simulink model "Three_ph_T_DDparam1"  (R2024b)
settings: Solver=VariableStepAuto  StartTime=0.0  StopTime=10  RelTol=1e-3
values from neighbouring files (symbols this model uses):
  Lp = 0    [Three_ph_TFimptest_DD.m]
  Ls = 0.084225    [Three_ph_TFimptest_DD.m]
  P = 200e6    (= 200000000)    [Three_ph_TFimptest_DD.m]
  Rp = 4.3218    [Three_ph_TFimptest_DD.m]
  Rs = 0.7938    [Three_ph_TFimptest_DD.m]
  V = 20e3    (= 20000)    [Three_ph_TFimptest_DD.m]
  V1 = 2 * V2    (= 20000)    [Three_ph_TFimptest_DD.m]
  V2 = 1e4    (= 10000)    [Three_ph_TFimptest_DD.m]
undefined symbols (not defined in the file or in its folder): D1, Delta
libraries: spsGroundLib x7, spsCurrentMeasurementLib x6, spsACVoltageSourceLib x3, spsLinearTransformerLib x3, spsVoltageMeasurementLib x3, spsThreePhaseVIMeasurementLib x2, spsThreePhaseTransformerTwoWindingsLib x1, spsThreePhaseProgrammableVoltageSourceLib x1, spspowerguiLib x1
settings Model: PacingRate=0.100000  Creator=salsarayreh  LastModifiedBy=PC1

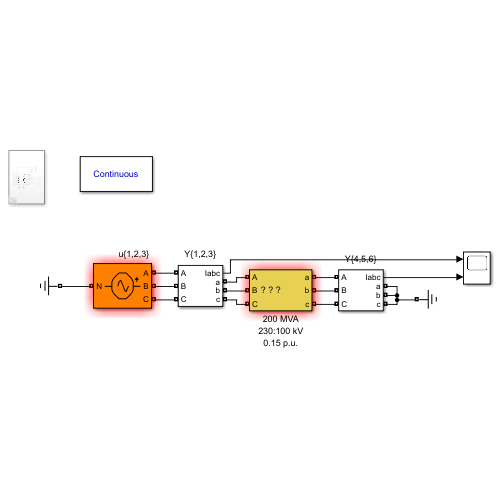
[thumbnail: Simulink's stored preview of the top-level diagram]
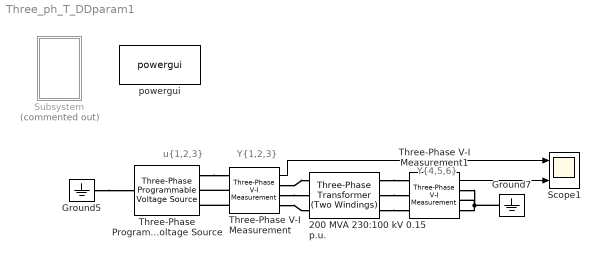
== system Three_ph_T_DDparam1 ==
  note: Y{4,5,6}
  note: Y{1,2,3}
  note: u{1,2,3}
  200 MVA 230:100 kV 0.15 p.u. : spsThreePhaseTransformerTwoWindingsLib/Three-Phase Transformer (Two Windings)  Winding1Connection=Delta (D1)  Winding2Connection=Delta (D1)  CoreType=Three single-phase transformers  SetSaturation=off  Hysteresis=off  DataFile='hysteresis'  SetInitialFlux=off  Measurements=All measurements (V I Fluxes)  UNITS=SI  NominalPower=[P , 50]  Winding1=[V1 Rp Lp ]  Winding2=[V2 Rs Ls]  Rm=Rm  Lm=Lm  L0=0.5  Saturation=[0 0;9.3114 683.7;785.26 875.13]  InitialFluxes=[-1.03850588171453 0.527233233676132 0.511272648041703]  BreakLoop=off  DiscreteSolver=Trapezoidal iterative  DataType=on  TransfoNumber=0
  Ground5 : spsGroundLib/Ground  LConnTagsString=a
  Ground7 : spsGroundLib/Ground  LConnTagsString=a
  Scope1 : Scope  NumInputPorts=2
  Subsystem : Subsystem  Commented=on
  Three-Phase Programmable Voltage Source : spsThreePhaseProgrammableVoltageSourceLib/Three-Phase Programmable Voltage Source  PositiveSequence="[V  0  50]"  VariationEntity=Amplitude  VariationType=Step  VariationTypeAlt=Step  VariationStep=-0.1  VariationRate=10  VariationMagnitude=0.3  VariationFrequency=2  VariationTiming="[0  0.14] + 1.5"  VariationPhaseA=off  Amplitudes=[1 0.8 1.2 1.0]  TimeValues=[0 0.1 0.15 0.2]  HarmonicGeneration=off  HarmonicA="[2 0.10  0  2]"  HarmonicB="[2  0  35 2]"  Timing="[1.2  99]"  BusType=swing  Pref=0  Qref=0  Qmin=-inf  Qmax=inf
  Three-Phase V-I Measurement : spsThreePhaseVIMeasurementLib/Three-Phase V-I Measurement  VoltageMeasurement=no  SetLabelV=off  LabelV=Vabc  Vpu=off  VpuLL=off  CurrentMeasurement=yes  SetLabelI=off  LabelI=Iabc  Ipu=off  Pbase=100e6  Vbase=500e3  OutputType=Complex  PhasorSimulation=off  PSBequivalent=0
  Three-Phase V-I Measurement1 : spsThreePhaseVIMeasurementLib/Three-Phase V-I Measurement  VoltageMeasurement=no  SetLabelV=off  LabelV=Vabc  Vpu=off  VpuLL=off  CurrentMeasurement=yes  SetLabelI=off  LabelI=Iabc  Ipu=off  Pbase=100e6  Vbase=500e3  OutputType=Complex  PhasorSimulation=off  PSBequivalent=0
  powergui : spspowerguiLib/powergui  Priority=1  SimulationMode=Continuous  SampleTime=50e-6  frequency=60  Iterations=50  frequencyindice=50  Pbase=100e6  ErrMax=1e-4  UnitsV=kV  UnitsW=MW  buscounter=0  FunctionMessages=off  echomessages=off  EnableUseOfTLC=off  CurrentSourceSwitches=off  DisableSnubberDevices=off  DisableRonSwitches=off  DisableVfSwitches=off  DisplayEquations=off  AutomaticDiscreteSolvers=off  SolverType=Tustin/Backward Euler (TBE)  Interpol=off  ExternalGateDelay=off  methode=off  Ts=100  x0status=blocks  SPID=on  SwTol=0  HookPort=off  NonlinearTolerance=1e-4  nMaxIteration=100  ContinueOnMaxIteration=off  RestoreLinks=warning  ResistiveCurrentMeasurement=off  Frange=[0:2:500]  Ylog=off  Xlog=on  ShowGrid=off  save=off  variable=ZData  structure=0  ZoomFFT=off  StartTime=0.0  cycles=1  DisplayStyle=1  fundamental=60  FreqAxis=off  MaxFrequency=1000  frequencyindicesteady=1  RmsSteady=1  display=off
  wires:
  Three-Phase V-I Measurement1/1 -> Scope1/2
  Three-Phase V-I Measurement/1 -> Scope1/1
  connections:
  Ground5/LConn1 -- Three-Phase Programmable Voltage Source/LConn1
  200 MVA 230:100 kV 0.15 p.u./RConn1 -- Three-Phase V-I Measurement1/LConn1
  200 MVA 230:100 kV 0.15 p.u./RConn2 -- Three-Phase V-I Measurement1/LConn2
  200 MVA 230:100 kV 0.15 p.u./RConn3 -- Three-Phase V-I Measurement1/LConn3
  Ground7/LConn1 -- Three-Phase V-I Measurement1/RConn1 -- Three-Phase V-I Measurement1/RConn2 -- Three-Phase V-I Measurement1/RConn3
  Three-Phase V-I Measurement/RConn2 -- 200 MVA 230:100 kV 0.15 p.u./LConn2
  Three-Phase V-I Measurement/RConn3 -- 200 MVA 230:100 kV 0.15 p.u./LConn3
  Three-Phase V-I Measurement/RConn1 -- 200 MVA 230:100 kV 0.15 p.u./LConn1
  Three-Phase V-I Measurement/LConn3 -- Three-Phase Programmable Voltage Source/RConn3
  Three-Phase V-I Measurement/LConn2 -- Three-Phase Programmable Voltage Source/RConn2
  Three-Phase Programmable Voltage Source/RConn1 -- Three-Phase V-I Measurement/LConn1

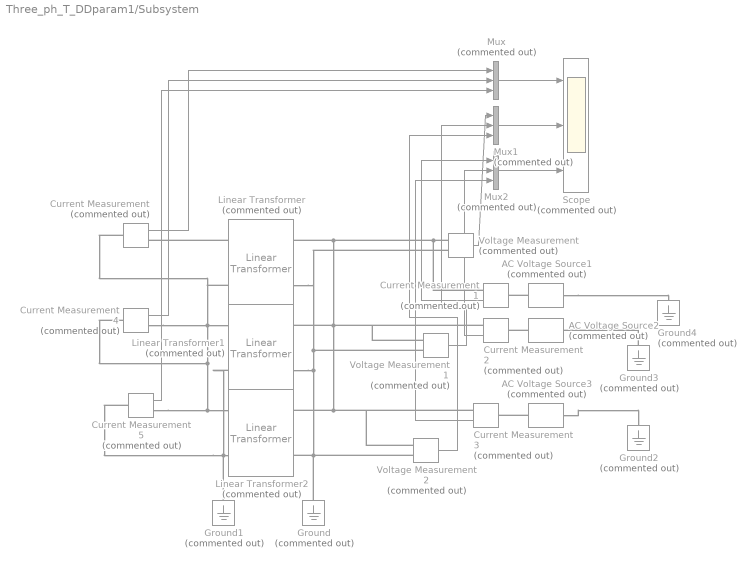
== system Three_ph_T_DDparam1/Subsystem ==
  AC Voltage Source1 : spsACVoltageSourceLib/AC Voltage Source  Commented=on  Amplitude=1  Phase=0  Frequency=50  SampleTime=0  Measurements=None  BusType=swing  Pref=10e3  Qref=0  Qmin=-inf  Qmax=+inf
  AC Voltage Source2 : spsACVoltageSourceLib/AC Voltage Source  Commented=on  Amplitude=1  Phase=-120  Frequency=50  SampleTime=0  Measurements=None  BusType=swing  Pref=10e3  Qref=0  Qmin=-inf  Qmax=+inf
  AC Voltage Source3 : spsACVoltageSourceLib/AC Voltage Source  Commented=on  Amplitude=1  Phase=120  Frequency=50  SampleTime=0  Measurements=None  BusType=swing  Pref=10e3  Qref=0  Qmin=-inf  Qmax=+inf
  Current Measurement{,1..5} (6 alike) : spsCurrentMeasurementLib/Current Measurement  Commented=on  PhasorSimulation=off  OutputType=Complex  PSBequivalent=0
  Ground{,1..4} (5 alike) : spsGroundLib/Ground  Commented=on  LConnTagsString=a
  Linear Transformer : spsLinearTransformerLib/Linear Transformer  Commented=on  UNITS=SI  NominalPower=[ 250e4 50 ]  winding1=[2e+05 4.3218 0.45856]  winding2=[1e+05 0.7938 0.084225]  ThreeWindings=off  winding3=[3.15e+05 0.7938 0.084225]  RmLm=[1.0804e+06 2e-3]  Measurements=All voltages and currents  DataType=on
  Linear Transformer1 : spsLinearTransformerLib/Linear Transformer  Commented=on  UNITS=SI  NominalPower=[ 250e4 50 ]  winding1=[2e+05 4.3218 0.45856]  winding2=[1e+05 0.7938 0.084225]  ThreeWindings=off  winding3=[3.15e+05 0.7938 0.084225]  RmLm=[1.0804e+06 2e-3]  Measurements=All voltages and currents  DataType=on
  Linear Transformer2 : spsLinearTransformerLib/Linear Transformer  Commented=on  UNITS=SI  NominalPower=[ 250e4 50 ]  winding1=[2e+05 4.3218 0.45856]  winding2=[1e+05 0.7938 0.084225]  ThreeWindings=off  winding3=[3.15e+05 0.7938 0.084225]  RmLm=[1.0804e+06 2e-3]  Measurements=All voltages and currents  DataType=on
  Mux : Mux  Commented=on  Inputs=3
  Mux1 : Mux  Commented=on  Inputs=3
  Mux2 : Mux  Commented=on  Inputs=3
  Scope : Scope  Commented=on  NumInputPorts=3
  Voltage Measurement : spsVoltageMeasurementLib/Voltage Measurement  Commented=on  PhasorSimulation=off  OutputType=Complex  PSBequivalent=0
  Voltage Measurement1 : spsVoltageMeasurementLib/Voltage Measurement  Commented=on  PhasorSimulation=off  OutputType=Complex  PSBequivalent=0
  Voltage Measurement2 : spsVoltageMeasurementLib/Voltage Measurement  Commented=on  PhasorSimulation=off  OutputType=Complex  PSBequivalent=0
  wires:
  Current Measurement4/1 -> Mux/2
  Voltage Measurement/1 -> Mux1/1
  Current Measurement/1 -> Mux/1
  Voltage Measurement2/1 -> Mux1/3
  Current Measurement5/1 -> Mux/3
  Mux1/1 -> Scope/2
  Current Measurement1/1 -> Mux2/1
  Current Measurement3/1 -> Mux2/3
  Voltage Measurement1/1 -> Mux1/2
  Current Measurement2/1 -> Mux2/2
  Mux2/1 -> Scope/3
  Mux/1 -> Scope/1
  connections:
  Current Measurement1/RConn1 -- Voltage Measurement1/LConn1 -- Current Measurement2/RConn1 -- Voltage Measurement2/LConn1 -- Current Measurement3/RConn1 -- Linear Transformer2/RConn1 -- Linear Transformer1/RConn1 -- Linear Transformer/RConn1 -- Voltage Measurement/LConn1
  Ground/LConn1 -- Voltage Measurement2/LConn2 -- Voltage Measurement1/LConn2 -- Voltage Measurement/LConn2 -- Linear Transformer/RConn2 -- Linear Transformer1/RConn2 -- Linear Transformer2/RConn2
  Ground1/LConn1 -- Current Measurement5/LConn1 -- Linear Transformer2/LConn2 -- Linear Transformer1/LConn2
  AC Voltage Source1/RConn1 -- Current Measurement1/LConn1
  Ground3/LConn1 -- AC Voltage Source2/LConn1
  Current Measurement4/RConn1 -- Current Measurement/LConn1 -- Linear Transformer/LConn2 -- Current Measurement5/RConn1 -- Linear Transformer2/LConn1 -- Current Measurement4/LConn1 -- Linear Transformer1/LConn1
  Linear Transformer/LConn1 -- Current Measurement/RConn1
  AC Voltage Source3/RConn1 -- Current Measurement3/LConn1
  AC Voltage Source1/LConn1 -- Ground4/LConn1
  AC Voltage Source3/LConn1 -- Ground2/LConn1
  AC Voltage Source2/RConn1 -- Current Measurement2/LConn1
